simulink model "test_overdrive"  (R2023b)
settings: Solver=VariableStepAuto  StartTime=0.0  StopTime=65  RelTol=1e-3
undefined symbols (not defined in the file or in its folder): DiscIntNeverNeededParam, dspDeleteFVToolLinkFromMask, gcbh
libraries: audiosources x2, audiomeasurements x2, simulink x2, dspsnks4 x1, dspfiltersrcs x1
settings Model: Creator=Thinkpad  LastModifiedBy=Thinkpad

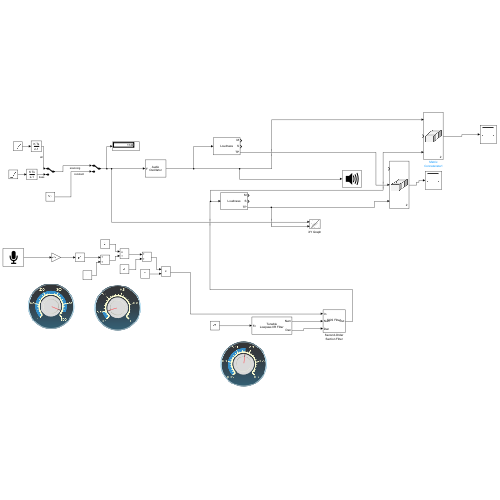
[thumbnail: Simulink's stored preview of the top-level diagram]
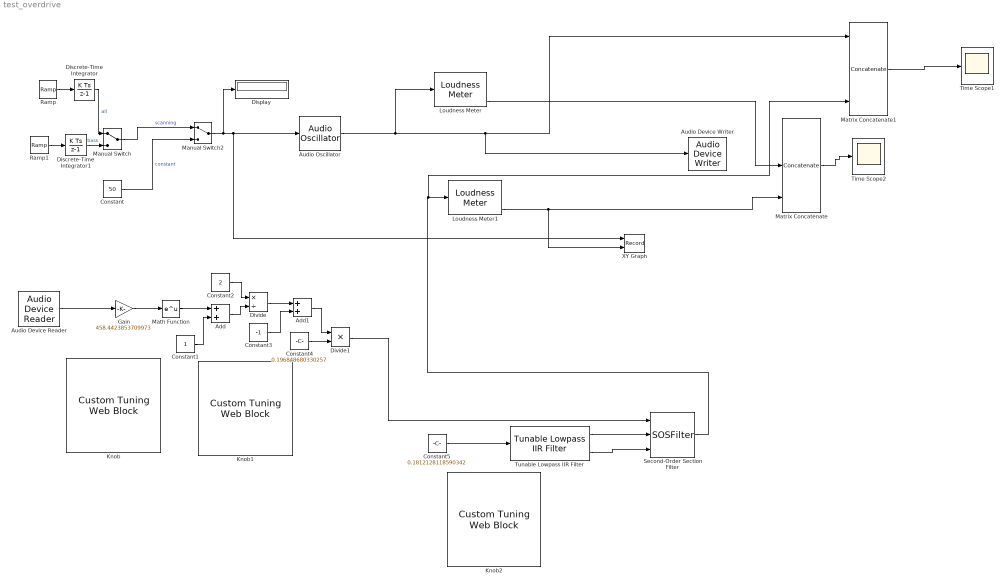
== system test_overdrive ==
  Add : Sum
  Add1 : Sum
  Audio Device Reader : audiosources/Audio Device Reader  Driver=DirectSound  Device=麦克风 (Scarlett 2i2 USB)  SampleRate=44100  NumChannels=1  SamplesPerFrame=4096  BitDepth=16-bit integer  NumBuffers=10  DefaultInputChannelMapping=on  InputChannelMapping=1:2  OutputNumOverrunSamples=off  OutputDataType=double  DriverIdx=1  DeviceWarnFlag=''
  Audio Device Writer : dspsnks4/Audio Device Writer  Driver=DirectSound  Device=扬声器 (Scarlett 2i2 USB)  InheritSampleRate=on  SampleRate=44100  BitDepth=16-bit integer  BufferSize=4096  NumBuffers=10  DefaultOutputChannelMapping=on  OutputChannelMapping=1:2  OutputNumUnderrunSamples=off  DriverIdx=1  DeviceWarnFlag=''
  Audio Oscillator : audiosources/Audio Oscillator  FrequencyPort=on  Frequency=1000  AmplitudePort=off  Amplitude=0.5  DCOffsetPort=off  PhaseOffset=0  DCOffset=0  WidthPort=off  Width=1  DutyCyclePort=off  DutyCycle=0.5  SampsPerFrame=4096  Fs=44100  OutputDataType=double  SimulateUsing=Code generation
      settings: SignalType=sine
  Constant : Constant  Value=50
  Constant1 : Constant
  Constant2 : Constant  Value=2
  Constant3 : Constant  Value=-1
  Constant4 : Constant  Value=0.196848680330257
  Constant5 : Constant  Value=0.1812128118590342
  Discrete-Time Integrator : DiscreteIntegrator  InitialCondition=10  SampleTime=-1  ICPrevOutput=DiscIntNeverNeededParam  ICPrevScaledInput=DiscIntNeverNeededParam
  Discrete-Time Integrator1 : DiscreteIntegrator  InitialCondition=10  SampleTime=-1  ICPrevOutput=DiscIntNeverNeededParam  ICPrevScaledInput=DiscIntNeverNeededParam
  Display : Display
  Divide : Product  Inputs=*/
  Divide1 : Product  Inputs=**
  Gain : Gain  Gain=458.4423853709973
  Knob : CustomTuningWebBlock  LabelPosition=Hide  ShowInitialText=on  Configuration="{\"components\":[{\"name\":\"CircularScaleComponent\",\"settings\":{\"bounds\":{\"max\":500,\"min\":1,\"tickInterval\":\"auto\"},\"direction\":\"cw\",\"flipLimits\":0,\"innerRadius\":0.6636618227670849,\"internalTickHeightScaleFactor\":1,\"labelColor\":[255,255,200],\"labelFont\":{\"font\":\"Arial\",\"fontSize\":12},\"labelRadius\":0.79,\"labelTransparency\":1,\"minorTickHeightScaleFactor\":0.2,\"needleImage\":{\"size\":[150,150],\"src\":\"data:image\\/svg+xml;base64,PD94bWwgdmVyc2lvbj0iMS4wIiBlbmNvZGluZz0idXRmLTgiPz4NCjwhLS0gR2VuZXJhdG9yOiBBZG9iZSBJbGx1c3RyYXRvciAyNS4yLjMsIFNWRyBFeHBvcnQgUGx1Zy1JbiAuIFNWRyBWZXJzaW9uOiA2LjAwIEJ1aWxkIDApICAtLT4NCjxzdmcgdmVyc2lvbj0iMS4xIiBpZD0iTGF5ZXJfMSIgeG1sbnM9Imh0dHA6Ly93d3cudzMub3JnLzIwMDAvc3ZnIiB4bWxuczp4bGluaz0iaHR0cDovL3d3dy53My5vcmcvMTk5OS94bGluayIgeD0iMHB4IiB5PSIwcHgiDQoJIHZpZXdCb3g9IjAgMCAxNTIgMTUyIiBzdHlsZT0iZW5hYmxl ...(+37472 chars)\"},\"needleOffset\":[0,0],\"needleOrientation\":-45,\"needleRotation\":90,\"needleSize\":{\"height\":0.44,\"width\":0.44},\"outerRadius\":0.5053386200069245,\"position\":[0,0,1,1],\"referencePoint\":\"auto\",\"scaleAngle\":270,\"scaleAngleOffset\":135,\"scaleColors\":[],\"scaleColorsSize\":0.2,\"scaleDirection\":\"CW\",\"scalePosition\":[0,0,1,1],\"showLabels\":1,\"showMinorTicks\":1,\"showSpanLine\":true,\"showTicks\":1,\"tickColor\":[252,252,197],\"tickTransparency\":1,\"valueBarColor\":[0,114,189],\"valueBarPosition\":[0,0,1,1],\"valueBarSize\":0.2,\"valueBarTransparency\":1}},{\"name\":\"BackgroundImageComponent\",\"settings\":{\"image\":{\"size\":[385,373],\"src\":\"data:image\\/svg+xml;base64,PD94bWwgdmVyc2lvbj0iMS4wIiBlbmNvZGluZz0idXRmLTgiPz4NCjwhLS0gR2VuZXJhdG9yOiBBZG9iZSBJbGx1c3RyYXRvciAyNS4wLjAsIFNWRyBFeHBvcnQgUGx1Zy1JbiAuIFNWRyBWZXJzaW9uOiA2LjAwIEJ1aWxkIDApICAtLT4NCjxzdmcgdmVyc2lvbj0iMS4xIg0KCSBpZD0iTGF5ZXJfMl8xXyIgeG1sbnM6Y2M9Imh0dHA6Ly9jcmVhdGl2ZWNvbW1vbnMub3JnL25zIyIgeG1sbnM6ZGM9Imh0dHA6Ly9wdXJsLm9yZy9kYy9lbGVtZW50cy8xLjEvIiB4bWxuczppbmtzY2FwZT0iaHR0cDovL3d3dy5pbmtzY2FwZS5vcmcv ...(+4184 chars)\",\"srcOrientation\":\"horizontal\"},\"position\":[0,0,1,1],\"scaleMode\":\"0\"}},{\"name\":\"ForegroundImageComponent\",\"settings\":{\"image\":{\"size\":[0,0],\"src\":\"default\",\"srcOrientation\":[]},\"isForeground\":1,\"position\":[0,0,1,1],\"scaleMode\":\"0\"}}],\"settings\":{\"BindingType\":\"param\",\"aspectRatio\":1,\"backgroundColor\":[0,0,0,\"1\"],\"backgroundOffset\":1,\"backgroundOpacity\":1,\"direction\":\"cw\",\"fixedAspectRatio\":\"on\",\"flipLimits\":0,\"foregroundColor\":[252,252,196],\"orientation\":\"horizontal\",\"showBackgroundColor\":false,\"value\":0,\"version\":\"R2023a\"},\"type\":\"CircularGauge\"}"
  Knob1 : CustomTuningWebBlock  LabelPosition=Hide  ShowInitialText=on  Configuration="{\"components\":[{\"name\":\"CircularScaleComponent\",\"settings\":{\"bounds\":{\"max\":1,\"min\":0.1,\"tickInterval\":\"auto\"},\"direction\":\"cw\",\"flipLimits\":0,\"innerRadius\":0.6636618227670849,\"internalTickHeightScaleFactor\":1,\"labelColor\":[255,255,200],\"labelFont\":{\"font\":\"Arial\",\"fontSize\":12},\"labelRadius\":0.79,\"labelTransparency\":1,\"minorTickHeightScaleFactor\":0.2,\"needleImage\":{\"size\":[150,150],\"src\":\"data:image\\/svg+xml;base64,PD94bWwgdmVyc2lvbj0iMS4wIiBlbmNvZGluZz0idXRmLTgiPz4NCjwhLS0gR2VuZXJhdG9yOiBBZG9iZSBJbGx1c3RyYXRvciAyNS4yLjMsIFNWRyBFeHBvcnQgUGx1Zy1JbiAuIFNWRyBWZXJzaW9uOiA2LjAwIEJ1aWxkIDApICAtLT4NCjxzdmcgdmVyc2lvbj0iMS4xIiBpZD0iTGF5ZXJfMSIgeG1sbnM9Imh0dHA6Ly93d3cudzMub3JnLzIwMDAvc3ZnIiB4bWxuczp4bGluaz0iaHR0cDovL3d3dy53My5vcmcvMTk5OS94bGluayIgeD0iMHB4IiB5PSIwcHgiDQoJIHZpZXdCb3g9IjAgMCAxNTIgMTUyIiBzdHlsZT0iZW5hYmxl ...(+37472 chars)\"},\"needleOffset\":[0,0],\"needleOrientation\":-45,\"needleRotation\":90,\"needleSize\":{\"height\":0.44,\"width\":0.44},\"outerRadius\":0.5053386200069245,\"position\":[0,0,1,1],\"referencePoint\":\"auto\",\"scaleAngle\":270,\"scaleAngleOffset\":135,\"scaleColors\":[],\"scaleColorsSize\":0.2,\"scaleDirection\":\"CW\",\"scalePosition\":[0,0,1,1],\"showLabels\":1,\"showMinorTicks\":1,\"showSpanLine\":true,\"showTicks\":1,\"tickColor\":[252,252,197],\"tickTransparency\":1,\"valueBarColor\":[0,114,189],\"valueBarPosition\":[0,0,1,1],\"valueBarSize\":0.2,\"valueBarTransparency\":1}},{\"name\":\"BackgroundImageComponent\",\"settings\":{\"image\":{\"size\":[385,373],\"src\":\"data:image\\/svg+xml;base64,PD94bWwgdmVyc2lvbj0iMS4wIiBlbmNvZGluZz0idXRmLTgiPz4NCjwhLS0gR2VuZXJhdG9yOiBBZG9iZSBJbGx1c3RyYXRvciAyNS4wLjAsIFNWRyBFeHBvcnQgUGx1Zy1JbiAuIFNWRyBWZXJzaW9uOiA2LjAwIEJ1aWxkIDApICAtLT4NCjxzdmcgdmVyc2lvbj0iMS4xIg0KCSBpZD0iTGF5ZXJfMl8xXyIgeG1sbnM6Y2M9Imh0dHA6Ly9jcmVhdGl2ZWNvbW1vbnMub3JnL25zIyIgeG1sbnM6ZGM9Imh0dHA6Ly9wdXJsLm9yZy9kYy9lbGVtZW50cy8xLjEvIiB4bWxuczppbmtzY2FwZT0iaHR0cDovL3d3dy5pbmtzY2FwZS5vcmcv ...(+4184 chars)\",\"srcOrientation\":\"horizontal\"},\"position\":[0,0,1,1],\"scaleMode\":\"0\"}},{\"name\":\"ForegroundImageComponent\",\"settings\":{\"image\":{\"size\":[0,0],\"src\":\"default\",\"srcOrientation\":[]},\"isForeground\":1,\"position\":[0,0,1,1],\"scaleMode\":\"0\"}}],\"settings\":{\"BindingType\":\"param\",\"aspectRatio\":1,\"backgroundColor\":[0,0,0,\"1\"],\"backgroundOffset\":1,\"backgroundOpacity\":1,\"direction\":\"cw\",\"fixedAspectRatio\":\"on\",\"flipLimits\":0,\"foregroundColor\":[252,252,196],\"orientation\":\"horizontal\",\"showBackgroundColor\":false,\"value\":0,\"version\":\"R2023a\"},\"type\":\"CircularGauge\"}"
  Knob2 : CustomTuningWebBlock  LabelPosition=Hide  ShowInitialText=on  Configuration="{\"components\":[{\"name\":\"CircularScaleComponent\",\"settings\":{\"bounds\":{\"max\":0.3,\"min\":0.05,\"tickInterval\":\"auto\"},\"direction\":\"cw\",\"flipLimits\":0,\"innerRadius\":0.6636618227670849,\"internalTickHeightScaleFactor\":1,\"labelColor\":[255,255,200],\"labelFont\":{\"font\":\"Arial\",\"fontSize\":12},\"labelRadius\":0.79,\"labelTransparency\":1,\"minorTickHeightScaleFactor\":0.2,\"needleImage\":{\"size\":[150,150],\"src\":\"data:image\\/svg+xml;base64,PD94bWwgdmVyc2lvbj0iMS4wIiBlbmNvZGluZz0idXRmLTgiPz4NCjwhLS0gR2VuZXJhdG9yOiBBZG9iZSBJbGx1c3RyYXRvciAyNS4yLjMsIFNWRyBFeHBvcnQgUGx1Zy1JbiAuIFNWRyBWZXJzaW9uOiA2LjAwIEJ1aWxkIDApICAtLT4NCjxzdmcgdmVyc2lvbj0iMS4xIiBpZD0iTGF5ZXJfMSIgeG1sbnM9Imh0dHA6Ly93d3cudzMub3JnLzIwMDAvc3ZnIiB4bWxuczp4bGluaz0iaHR0cDovL3d3dy53My5vcmcvMTk5OS94bGluayIgeD0iMHB4IiB5PSIwcHgiDQoJIHZpZXdCb3g9IjAgMCAxNTIgMTUyIiBzdHlsZT0iZW5hYmxl ...(+37472 chars)\"},\"needleOffset\":[0,0],\"needleOrientation\":-45,\"needleRotation\":90,\"needleSize\":{\"height\":0.44,\"width\":0.44},\"outerRadius\":0.5053386200069245,\"position\":[0,0,1,1],\"referencePoint\":\"auto\",\"scaleAngle\":270,\"scaleAngleOffset\":135,\"scaleColors\":[],\"scaleColorsSize\":0.2,\"scaleDirection\":\"CW\",\"scalePosition\":[0,0,1,1],\"showLabels\":1,\"showMinorTicks\":1,\"showSpanLine\":true,\"showTicks\":1,\"tickColor\":[252,252,197],\"tickTransparency\":1,\"valueBarColor\":[0,114,189],\"valueBarPosition\":[0,0,1,1],\"valueBarSize\":0.2,\"valueBarTransparency\":1}},{\"name\":\"BackgroundImageComponent\",\"settings\":{\"image\":{\"size\":[385,373],\"src\":\"data:image\\/svg+xml;base64,PD94bWwgdmVyc2lvbj0iMS4wIiBlbmNvZGluZz0idXRmLTgiPz4NCjwhLS0gR2VuZXJhdG9yOiBBZG9iZSBJbGx1c3RyYXRvciAyNS4wLjAsIFNWRyBFeHBvcnQgUGx1Zy1JbiAuIFNWRyBWZXJzaW9uOiA2LjAwIEJ1aWxkIDApICAtLT4NCjxzdmcgdmVyc2lvbj0iMS4xIg0KCSBpZD0iTGF5ZXJfMl8xXyIgeG1sbnM6Y2M9Imh0dHA6Ly9jcmVhdGl2ZWNvbW1vbnMub3JnL25zIyIgeG1sbnM6ZGM9Imh0dHA6Ly9wdXJsLm9yZy9kYy9lbGVtZW50cy8xLjEvIiB4bWxuczppbmtzY2FwZT0iaHR0cDovL3d3dy5pbmtzY2FwZS5vcmcv ...(+4184 chars)\",\"srcOrientation\":\"horizontal\"},\"position\":[0,0,1,1],\"scaleMode\":\"0\"}},{\"name\":\"ForegroundImageComponent\",\"settings\":{\"image\":{\"size\":[0,0],\"src\":\"default\",\"srcOrientation\":[]},\"isForeground\":1,\"position\":[0,0,1,1],\"scaleMode\":\"0\"}}],\"settings\":{\"BindingType\":\"param\",\"aspectRatio\":1,\"backgroundColor\":[0,0,0,\"1\"],\"backgroundOffset\":1,\"backgroundOpacity\":1,\"direction\":\"cw\",\"fixedAspectRatio\":\"on\",\"flipLimits\":0,\"foregroundColor\":[252,252,196],\"orientation\":\"horizontal\",\"showBackgroundColor\":false,\"value\":0,\"version\":\"R2023a\"},\"type\":\"CircularGauge\"}"
  Loudness Meter : audiomeasurements/Loudness Meter  ChannelWeights=[ 1, 1, 1, 1.41, 1.41 ]  UseRelativeScale=off  TargetLoudness=-23.0  OutputTruePeak=on  InheritSampleRate=on  SampleRate=44100  SimulateUsing=Code generation
  Loudness Meter1 : audiomeasurements/Loudness Meter  ChannelWeights=[ 1, 1, 1, 1.41, 1.41 ]  UseRelativeScale=off  TargetLoudness=-23.0  OutputTruePeak=on  InheritSampleRate=on  SampleRate=44100  SimulateUsing=Code generation
  Manual Switch : ManualSwitch
  Manual Switch2 : ManualSwitch
  Math Function : Math  OutputSignalType=real
  Matrix Concatenate : Concatenate  NumInputs=3  Mode=Multidimensional array  ConcatenateDimension=2
  Matrix Concatenate1 : Concatenate  NumInputs=3  Mode=Multidimensional array  ConcatenateDimension=2
  Ramp : simulink/Sources/Ramp  slope=10  start=0  InitialOutput=0
  Ramp1 : simulink/Sources/Ramp  slope=1  start=0  InitialOutput=0
  Second-Order Section Filter : SOSFilter  LoadFcn=dspDeleteFVToolLinkFromMask(gcbh);  FilterStructure=Direct form II  CoeffSource=Input ports
      settings: DeleteFcn=dspLinkFVTool2Mask(gcbh,'close')  ModelCloseFcn=dspLinkFVTool2Mask(gcbh,'close')  PreSaveFcn=dspUnlinkFVToolFromMask(gcbh);  PostSaveFcn=dspRestoreLinkFVTool2Mask(gcbh);  CloseFcn=dspLinkFVTool2Mask(gcbh,'close')  InputPortMap=u0,u1,u2
      settings: CopyFcn=|
      | ud = get_param(gcbh,'UserData');
      | if isfield(ud,'fvtool')
      |   ud = rmfield(ud,'fvtool');
      |   set_param(gcbh,'UserData',ud);
      | end
      | clear ud
  Time Scope1 : Scope
  Time Scope2 : Scope
  Tunable Lowpass IIR Filter : dspfiltersrcs/Tunable Lowpass IIR Filter  DesignMethod=Butterworth  FilterOrderPort=off  FilterOrder=6  MaxOrder=10  HasScaleValues=off  F3dBPort=on  F3dB=0.25  ApassPort=off  Apass=1  AstopPort=off  Astop=60  SampleTime=-1  OutputDataType=double  SimulateUsing=Code generation
  XY Graph : Record  FileSettingsInternal="{\"entries\":[{\"content\":{\"excelSettings\":{\"content\":{},\"type\":\"Streamout.ExcelSettings\"}},\"type\":\"Streamout.FileSettingStorage\",\"uuid\":\"\"}],\"packageUris\":[\"http:\\/\\/schema.mathworks.com\\/mf0\\/streamout_blocks\\/R2020a\"],\"version\":\"1.0\"}"  Layout=[1 1]  SignalsInternal="{\"entries\":[{\"content\":{\"signals\":[{\"content\":{\"blockPath\":[],\"dimensions\":[1],\"domain\":\"\",\"lineColor\":\"#0072bd\",\"plots\":[1],\"port\":1,\"sid\":[\"\"],\"signalID\":35170,\"signalName\":\"Manual Switch2\"},\"type\":\"RecordBlkView.Signal\",\"uuid\":\"\"},{\"content\":{\"blockPath\":[],\"dimensions\":[1,1],\"domain\":\"\",\"lineColor\":\"#d95319\",\"plots\":[1],\"port\":2,\"sid\":[\"\"],\"signalID\":35174,\"signalName\":\"Loudness Meter1:3\"},\"type\":\"RecordBlkView.Signal\",\"uuid\":\"\"}]},\"type\":\"RecordBlkView.InputSignals\",\"uuid\":\"\"}],\"packageUris\":[\"http:\\/\\/schema.mathworks.com\\/mf0\\/streamout_blocks\\/R2020a\"],\"version\":\"1.0\"}"  VisualizationBindings="{\"xyplotplugin\":{\"info\":[{\"series\":[{\"bindingParametersList\":[{\"parameter\":\"X-Axis\",\"signalID\":35170,\"signalName\":\"Manual Switch2\"},{\"parameter\":\"Y-Axis\",\"signalID\":35174,\"signalName\":\"Loudness Meter1:3\"}],\"seriesID\":2193}],\"subplotID\":1}]}}"  CompatibilityTag=XY
  wires:
  Manual Switch/1 -> Manual Switch2/1  "scanning"
  Constant/1 -> Manual Switch2/2  "constant"
  Discrete-Time Integrator/1 -> Manual Switch/1  "all"
  Discrete-Time Integrator1/1 -> Manual Switch/2  "bass"
  Ramp1/1 -> Discrete-Time Integrator1/1
  Loudness Meter1/3 -> XY Graph/2, Matrix Concatenate/3
  Ramp/1 -> Discrete-Time Integrator/1
  Matrix Concatenate1/1 -> Time Scope1/1
  Matrix Concatenate/1 -> Time Scope2/1
  Audio Oscillator/1 -> Loudness Meter/1, Matrix Concatenate1/1, Audio Device Writer/1
  Loudness Meter/3 -> Matrix Concatenate/2
  Manual Switch2/1 -> Display/1, Audio Oscillator/1, XY Graph/1
  Audio Device Reader/1 -> Gain/1
  Gain/1 -> Math Function/1
  Math Function/1 -> Add/1
  Constant1/1 -> Add/2
  Add/1 -> Divide/2
  Constant2/1 -> Divide/1
  Divide/1 -> Add1/1
  Constant3/1 -> Add1/2
  Add1/1 -> Divide1/1
  Constant4/1 -> Divide1/2
  Second-Order Section Filter/1 -> Matrix Concatenate1/3, Loudness Meter1/1
  Tunable Lowpass IIR Filter/1 -> Second-Order Section Filter/2
  Divide1/1 -> Second-Order Section Filter/1
  Tunable Lowpass IIR Filter/2 -> Second-Order Section Filter/3
  Constant5/1 -> Tunable Lowpass IIR Filter/1
